simulink model "exper_2"  (Simulink 7.3)
settings: Solver=ode45  StartTime=0.0  StopTime=10.0  RelTol=1e-3
settings Model: Creator=Administrator  LastModifiedBy=Administrator

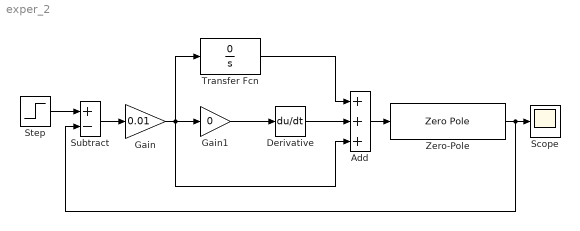
== system exper_2 ==
  Add : Sum  Inputs=+++  OutDataType=fixdt(1, 16)  OutScaling=2^-10
  Derivative : Derivative
  Gain : Gain  Gain=0.01  ParameterDataType=fixdt(1, 16)  ParameterScaling=2^0  OutDataType=fixdt(1, 16)  OutScaling=2^0
  Gain1 : Gain  Gain=0  ParameterDataType=fixdt(1, 16)  ParameterScaling=2^0  OutDataType=fixdt(1, 16)  OutScaling=2^0
  Scope : Scope
  Step : Step  SampleTime=0
  Subtract : Sum  Inputs=+-  OutDataType=fixdt(1, 16)  OutScaling=2^-10
  Transfer Fcn : TransferFcn  Numerator=[0]  Denominator=[1 0]
  Zero-Pole : ZeroPole  Zeros=[ ]  Poles=[0 -3 -1 -1]
  wires:
  Step/1 -> Subtract/1
  Subtract/1 -> Gain/1
  Gain/1 -> Gain1/1, Transfer Fcn/1, Add/3
  Gain1/1 -> Derivative/1
  Derivative/1 -> Add/2
  Transfer Fcn/1 -> Add/1
  Add/1 -> Zero-Pole/1
  Zero-Pole/1 -> Scope/1, Subtract/2
